simulink model "ToneGenerator"  (R2026a)
settings: Solver=VariableStepAuto  StopTime=.001
libraries: dsphdlsigops2 x1
settings Model: Creator=vijayenk  LastModifiedBy=vijayenk

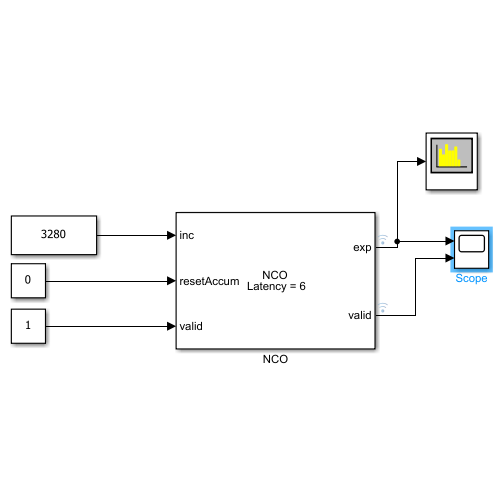
[thumbnail: Simulink's stored preview of the top-level diagram]
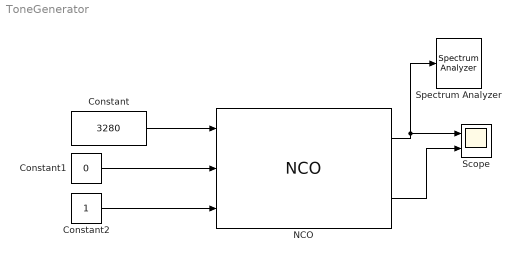
== system ToneGenerator ==
  Constant : Constant  Value=3280  OutDataTypeStr=uint32  SampleTime=1/200e6
  Constant1 : Constant  Value=0  OutDataTypeStr=boolean  SampleTime=1/200e6
  Constant2 : Constant  OutDataTypeStr=boolean  SampleTime=1/200e6
  NCO : dsphdlsigops2/NCO  PhaseIncrementSource=Input port  PhaseIncrement=100  Frequency=510  FreqResolution=0.05  SamplingFreq=4000  PhaseOffsetSource=Property  PhaseOffset=0  PhaseOffsetR=pi/3  DitherSource=Property  NumDitherBits=4  SamplesPerFrame=1  LUTCompress=off  ResetAction=on  Waveform=Complex exponential  PhasePort=off  SimulateUsing=Code generation  AccumulatorWL=16  PhaseQuantization=on  NumQuantizerAccumulatorBits=12  OutputDataType=Binary point scaling  OutputWL=16  OutputFL=14
      settings: LibrarySourceBlock=dsphdlsrcs2/NCO
  Scope : Scope  NumInputPorts=2
      settings: ActiveDisplayYMinimum=-1.1392716535433072  ActiveDisplayYMaximum=1.3607283464566928
  Spectrum Analyzer : SpectrumAnalyzer  WindowPosition=[160.000000,211.000000,800.000000,500.000000,]  Visible=on  ScopeFrameLocation=window  WindowInvariantSamplesPerUpdate=on  Span=200000000  StartFrequency=-100000000  StopFrequency=100000000  YLimits=[-136.7901 48.4894]  SelectedToolstripTab=spectrumAnalyzerToolstrip.measurementsTab
  wires:
  Constant/1 -> NCO/1
  Constant1/1 -> NCO/2
  Constant2/1 -> NCO/3
  NCO/2 -> Scope/2
  NCO/1 -> Scope/1, Spectrum Analyzer/1
